simulink model "controlled_system"  (R2024a)
settings: Solver=ode23s  StartTime=0.0  StopTime=70  FixedStep=1e-6  MaxStep=1e-3  RelTol=1e-3
values from neighbouring files (symbols this model uses):
  B = 0.068    [parameters.m]
  h = 0.009    [parameters.m]
  J = 0.51    [parameters.m]
  Ki = 5000    [parameters.m]
  Kp = 180    [parameters.m]
  Psisn = 1.48    [parameters.m]
  r = 4    [parameters.m]
  umax = 380    [parameters.m]
  umin = -umax    (= -380)    [parameters.m]
  Vac = 230    [parameters.m]
  wb = wn / np    (= 104.71975512)    [parameters.m]
libraries: DEMDlib x8, slpidlib x1, simulink x1
settings Model: Creator=roberto  LastModifiedBy=roberto
settings DebuggingCC: ReadBeforeWriteMsg=DisableAll  WriteAfterWriteMsg=DisableAll  WriteAfterReadMsg=DisableAll  MultiTaskDSMMsg=none
settings HardwareCC: ProdBitPerLong=64  ProdHWDeviceType=AMD->x86-64 (Linux 64)
settings ModelReferenceCC: UpdateModelReferenceTargets=IfOutOfDate
settings SFSimCC: SFSimEcho=off

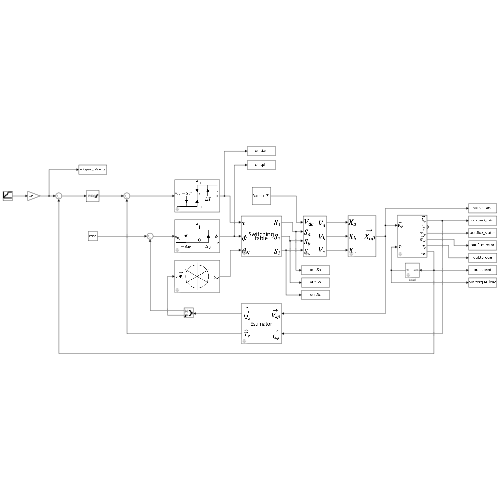
[thumbnail: Simulink's stored preview of the top-level diagram]
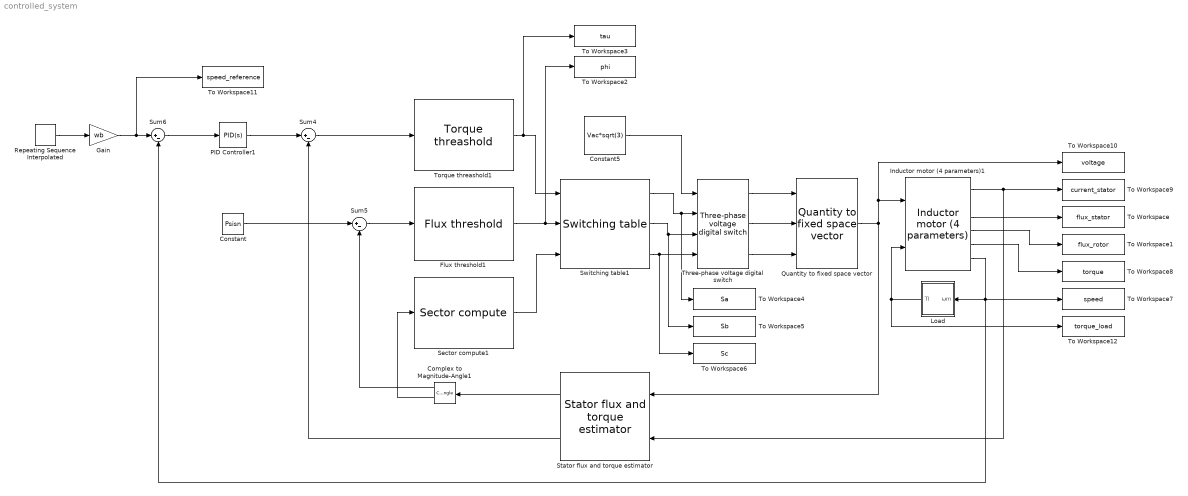
== system controlled_system ==
  Complex to Magnitude-Angle1 : ComplexToMagnitudeAngle
  Constant : Constant  Value=Psisn
  Constant5 : Constant  Value=Vac*sqrt(3)
  Flux threshold1 : DEMDlib/DTC/Flux threshold  dpsi=dPsi
      settings: SourceProductName=DEMD
  Gain : Gain  Gain=wb
  Inductor motor (4 parameters)1 : DEMDlib/Inductor motor (4 parameters)  Rs=Rs  Lks=Lks  Rr=Rkr  Lm=Lkm  np=np  J=J  B=B
      settings: SourceProductName=DEMD
  Load : Subsystem  mask(Quadratic load){r=r, k=h}
      mask DialogControl Control2 Prompt: Ratio (ωl/ωm)
      mask DialogControl Control2_copy Prompt: Load proportional coefficient (Nm s^2 / rad^2)
  PID Controller1 : slpidlib/PID Controller  Controller=PID  Form=Parallel  TimeDomain=Continuous-time  UseExternalTs=off  SampleTime=-1  IntegratorMethod=Forward Euler  FilterMethod=Forward Euler  ControllerParametersSource=internal  P=Kp  I=Ki  UseKiTs=off  D=0  UseExternalDerivativeSource=off  N=100  UseFilter=on  TunerSelectOption=Transfer Function Based (PID Tuner App)  InitialConditionSource=internal  InitialConditionForIntegrator=0  InitialConditionForFilter=0  DifferentiatorICPrevScaledInput=0  ExternalReset=none  TrackingMode=off  Kt=1  LimitOutput=on  SatLimitsSource=internal  UpperSaturationLimit=umax  LowerSaturationLimit=umin  LinearizeAsGain=on  AntiWindupMode=clamping  Kb=1  LimitIntegrator=off  UpperIntegratorSaturationLimit=inf  LowerIntegratorSaturationLimit=-inf  POutMin=[]  POutMax=[]  IOutMin=[]  IOutMax=[]  DOutMin=[]  DOutMax=[]  NOutMin=[]  NOutMax=[]  SumOutMin=[]  SumOutMax=[]  SaturationOutMin=[]  SaturationOutMax=[]  PParamMin=[]  PParamMax=[]  IParamMin=[]  IParamMax=[]  DParamMin=[]  DParamMax=[]  NParamMin=[]  NParamMax=[]  KbParamMin=[]  KbParamMax=[]  KtParamMin=[]  KtParamMax=[]  KbOutMin=[]  KbOutMax=[]  KtOutMin=[]  KtOutMax=[]  IntegratorOutMin=[]  IntegratorOutMax=[]  FilterOutMin=[]  FilterOutMax=[]  SumI1OutMin=[]  SumI1OutMax=[]  SumI2OutMin=[]  SumI2OutMax=[]  SumI3OutMin=[]  SumI3OutMax=[]  SumI4OutMin=[]  SumI4OutMax=[]  SumDOutMin=[]  SumDOutMax=[]  DifferentiatorOutMin=[]  DifferentiatorOutMax=[]  FilterDiffOutCoefMin=[]  FilterDiffOutCoefMax=[]  ReciprocalOutMin=[]  ReciprocalOutMax=[]  SumDenOutMin=[]  SumDenOutMax=[]  SumNumOutMin=[]  SumNumOutMax=[]  DivideOutMin=[]  DivideOutMax=[]  UdiffTsProdOutMin=[]  UdiffTsProdOutMax=[]  NTsProdOutMin=[]  NTsProdOutMax=[]  UintegralTsProdOutMin=[]  UintegralTsProdOutMax=[]  UngainTsProdOutMin=[]  UngainTsProdOutMax=[]  ClampingZeroOutDataTypeStr=Inherit: Inherit via back propagation  ClampingZeroOutMin=[]  ClampingZeroOutMax=[]  FilterDenConstantOutDataTypeStr=Inherit: Inherit via back propagation  FilterDenConstantOutMin=[]  FilterDenConstantOutMax=[]  PCopyOutDataTypeStr=Inherit: Inherit via back propagation  PCopyOutMin=[]  PCopyOutMax=[]  NCopyOutDataTypeStr=Inherit: Inherit via back propagation  NCopyOutMin=[]  NCopyOutMax=[]  IntegratorContinuousStateAttributes=''  IntegratorStateMustResolveToSignalObject=off  IntegratorRTWStateStorageClass=Auto  FilterContinuousStateAttributes=''  FilterStateMustResolveToSignalObject=off  FilterRTWStateStorageClass=Auto  ParallelPVariant=InternalParameters  IdealPVariant=Disabled  IVariant=InternalParameters  DVariant=InternalParameters  IntegratorVariant=Continuous  SatVariant=Enabled  AWVariant=ContClampingParallel  PCopyVariant=Disabled  TRVariant=Disabled  FdbkBlocksVariant=Forward  IdealPFdbkVariant=Disabled  SatFdbkVariant=Disabled  DerivativeFilterVariant=ContFilter  NVariant=InternalParameters  NCopyVariant=Disabled  FilterICVariant=InternalICsFilter  IntegratorICVariant=InternalICs  ExternalResetVariant=Disabled  TRSumVariant=Passthrough  SumFdbkVariant=Disabled  SumVariant=Sum_PID  TsampFilterVariant=InternalTs  TsampNgainVariant=Passthrough  TsampIntegralVariant=Disabled_SignalSpec  ExternalSaturationOutDataTypeStr=Inherit: Same as second input  DerivativeSourceVariant=ErrorSignal
  Quantity to fixed space vector : DEMDlib/Quantity to fixed space vector
      settings: SourceProductName=DEMD
  Repeating Sequence Interpolated : simulink/Sources/Repeating Sequence Interpolated  OutValues=[0 0.1 0.1 0.2 0.2].'  TimeValues=[0 20 30 40 70].'  LookUpMeth=Interpolation-Use End Values  tsamp=0.01  OutMin=[]  OutMax=[]  OutDataTypeStr=double  OutputDataTypeScalingMode=double  OutDataType=fixdt(0,8)  OutScaling=2^-10
  Sector compute1 : DEMDlib/DTC/Sector compute
      settings: SourceProductName=DEMD
  Stator flux and torque estimator : DEMDlib/DTC/Stator flux and torque estimator  Rs=Rs  Lks=Lks  np=np  a=alpha
      settings: SourceProductName=DEMD
  Sum4 : Sum  Inputs=|+-
  Sum5 : Sum  Inputs=|+-
  Sum6 : Sum  Inputs=|+-
  Switching table1 : DEMDlib/DTC/Switching table
      settings: SourceProductName=DEMD
  Three-phase voltage digital switch : DEMDlib/Three-phase voltage digital switch
      settings: SourceProductName=DEMD
  To Workspace : ToWorkspace  VariableName=flux_stator  SaveFormat=Timeseries  SampleTime=-1
  To Workspace1 : ToWorkspace  VariableName=flux_rotor  SaveFormat=Timeseries  SampleTime=-1
  To Workspace10 : ToWorkspace  VariableName=voltage  SaveFormat=Timeseries  SampleTime=-1
  To Workspace11 : ToWorkspace  VariableName=speed_reference  SaveFormat=Timeseries  SampleTime=-1
  To Workspace12 : ToWorkspace  VariableName=torque_load  SaveFormat=Timeseries  SampleTime=-1
  To Workspace2 : ToWorkspace  VariableName=phi  SaveFormat=Timeseries  SampleTime=-1
  To Workspace3 : ToWorkspace  VariableName=tau  SaveFormat=Timeseries  SampleTime=-1
  To Workspace4 : ToWorkspace  VariableName=Sa  SaveFormat=Timeseries  SampleTime=-1
  To Workspace5 : ToWorkspace  VariableName=Sb  SaveFormat=Timeseries  SampleTime=-1
  To Workspace6 : ToWorkspace  VariableName=Sc  SaveFormat=Timeseries  SampleTime=-1
  To Workspace7 : ToWorkspace  VariableName=speed  SaveFormat=Timeseries  SampleTime=-1
  To Workspace8 : ToWorkspace  VariableName=torque  SaveFormat=Timeseries  SampleTime=-1
  To Workspace9 : ToWorkspace  VariableName=current_stator  SaveFormat=Timeseries  SampleTime=-1
  Torque threashold1 : DEMDlib/DTC/Torque threashold  dT=dT
      settings: SourceProductName=DEMD
  wires:
  Inductor motor (4 parameters)1/6 -> To Workspace7/1, Sum6/2, Load/1(ωm)
  Load/1(Tl) -> Inductor motor (4 parameters)1/2, To Workspace12/1
  Quantity to fixed space vector/1 -> Inductor motor (4 parameters)1/1, To Workspace10/1, Stator flux and torque estimator/1
  Sector compute1/1 -> Switching table1/3
  Flux threshold1/1 -> To Workspace2/1, Switching table1/2
  Constant/1 -> Sum5/1
  Inductor motor (4 parameters)1/1 -> To Workspace9/1, Stator flux and torque estimator/2
  Stator flux and torque estimator/1 -> Complex to Magnitude-Angle1/1
  Complex to Magnitude-Angle1/1 -> Sum5/2
  Complex to Magnitude-Angle1/2 -> Sector compute1/1
  Stator flux and torque estimator/2 -> Sum4/2
  Switching table1/3 -> To Workspace6/1, Three-phase voltage digital switch/4
  Switching table1/2 -> To Workspace5/1, Three-phase voltage digital switch/3
  Switching table1/1 -> Three-phase voltage digital switch/2, To Workspace4/1
  Constant5/1 -> Three-phase voltage digital switch/1
  Three-phase voltage digital switch/1 -> Quantity to fixed space vector/1
  Three-phase voltage digital switch/2 -> Quantity to fixed space vector/2
  Three-phase voltage digital switch/3 -> Quantity to fixed space vector/3
  Inductor motor (4 parameters)1/3 -> To Workspace/1
  Inductor motor (4 parameters)1/4 -> To Workspace1/1
  Repeating Sequence Interpolated/1 -> Gain/1
  Torque threashold1/1 -> To Workspace3/1, Switching table1/1
  Sum5/1 -> Flux threshold1/1
  Sum4/1 -> Torque threashold1/1
  Sum6/1 -> PID Controller1/1
  PID Controller1/1 -> Sum4/1
  Gain/1 -> Sum6/1, To Workspace11/1
  Inductor motor (4 parameters)1/5 -> To Workspace8/1

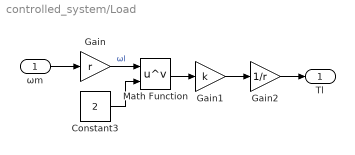
== system controlled_system/Load ==
  ωm : Inport
  Constant3 : Constant  Value=2
  Gain : Gain  Gain=r
  Gain1 : Gain  Gain=k
  Gain2 : Gain  Gain=1/r
  Math Function : Math  Operator=pow
  Tl : Outport
  wires:
  Gain/1 -> Math Function/1  "ωl"
  Constant3/1 -> Math Function/2
  Math Function/1 -> Gain1/1
  Gain1/1 -> Gain2/1
  Gain2/1 -> Tl/1
  ωm/1 -> Gain/1
